simulink model "QPSK_ad9361_radioIO_capture"  (R2017b)
settings: Solver=VariableStepAuto  StartTime=0.0  StopTime=inf  RelTol=1e-3  EnableMultiTasking=on
PreLoadFcn:
  | adi9361_preload(bdroot,'rx');
  | sdrqpsktx = sdrzqpsktxFMC234_init;
  | % sdrqpskrx = sdrzqpskrxFMC234_init;
  | sdrqpskrx = zynqRadioQPSKRxAD9361AD9364SL_init_2MSPS
InitFcn:
  | sdrqpsktx = sdrzqpsktxFMC234_init;
  | % sdrqpskrx = sdrzqpskrxFMC234_init;
  | sdrqpskrx = zynqRadioQPSKRxAD9361AD9364SL_init_2MSPS
undefined symbols (not defined in the file or in its folder): D, dBval, DCLeak_Matrix, designMultirateFIR, dfilt, fuzz_val, GainImb_Matrix, gcbh, IP2_Matrix, IP3_Matrix, magnitude, rcfiltgaincompat
libraries: simrfV2elements x12, simulink x7, dsparch4 x6, simrfV2util1 x4, fl_lib x4, dspmlti4 x3, simrfV2junction1 x3, commdigbbndpm3 x3, dspstat3 x3, dspobslib x3, simulink_extras x2, dspsigattribs x2
(part 2 of 3)

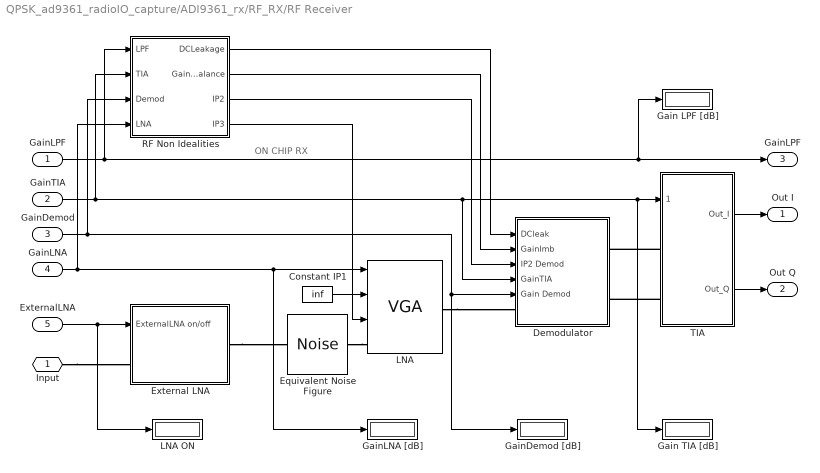
== system QPSK_ad9361_radioIO_capture/ADI9361_rx/RF_RX/RF Receiver ==
  note: ON CHIP RX
  GainLPF : Inport
  GainTIA : Inport  Port=2
  GainDemod : Inport  Port=3
  GainLNA : Inport  Port=4
  ExternalLNA : Inport  Port=5
  Constant IP1 : Constant  Value=inf
  Demodulator : Subsystem
  Equivalent Noise Figure : simrfV2sources1/Noise  SimulinkInputSignalType=Ideal voltage  NoiseType=White  NoisePSD=4*1.381e-23*290*50*10^(NF/10)  CarrierFreq=fc_RF Hz  InternalGrounding=off
      settings: SourceProductName=RF Blockset  SourceProductBaseCode=RB
  External LNA : Subsystem
  Gain LPF [dB] : Display
  Gain TIA [dB] : Display
  GainDemod [dB] : Display
  GainLNA [dB] : Display
  LNA : simrfV2elements/VGA  classname=vga  Zin=Rin  Zout=50  IO=Input  InternalGrounding=on
      settings: SourceProductName=RF Blockset  SourceProductBaseCode=RB
  LNA ON : Display
  RF Non Idealities : Subsystem
  TIA : Subsystem
  Input : PMIOPort  Port=1  Side=Left
  Out I : Outport
  Out Q : Outport  Port=2
  "GainLPF " : Outport  Port=3
  wires:
  GainTIA/1 -> RF Non Idealities/2(TIA), Gain TIA [dB]/1, TIA/1(Gain TIA), Demodulator/4(GainTIA)
  TIA/1(Out_I) -> Out I/1
  TIA/2(Out_Q) -> Out Q/1
  GainDemod/1 -> RF Non Idealities/3(Demod), Demodulator/5(Gain Demod), GainDemod [dB]/1
  GainLNA/1 -> LNA/1, GainLNA [dB]/1, RF Non Idealities/4(LNA)
  GainLPF/1 -> "GainLPF "/1, Gain LPF [dB]/1, RF Non Idealities/1(LPF)
  RF Non Idealities/1(DCLeakage) -> Demodulator/1(DCleak)
  RF Non Idealities/3(IP2) -> Demodulator/3(IP2 Demod)
  RF Non Idealities/4(IP3) -> LNA/3
  Constant IP1/1 -> LNA/2
  ExternalLNA/1 -> LNA ON/1, External LNA/1(ExternalLNA on/off)
  RF Non Idealities/2(GainImbalance) -> Demodulator/2(GainImb)
  connections:
  LNA/RConn1 -- Demodulator/LConn1
  TIA/LConn1 -- Demodulator/RConn1
  TIA/LConn2 -- Demodulator/RConn2
  Equivalent Noise Figure/LConn1 -- LNA/LConn1
  Input/RConn1 -- External LNA/LConn1
  External LNA/RConn1 -- Equivalent Noise Figure/RConn1

== system QPSK_ad9361_radioIO_capture/ADI9361_rx/Subsystem6/Subsystem1 ==
  Data Type Conversion : DataTypeConversion  OutDataTypeStr=boolean
  Pulse Generator2 : DiscretePulseGenerator  SampleTime=Trf
  START : Outport
  wires:
  Pulse Generator2/1 -> Data Type Conversion/1
  Data Type Conversion/1 -> START/1

== system QPSK_ad9361_radioIO_capture/ADI9361_rx/Subsystem6/Subsystem2 ==
  s : Inport
  w : Inport  Port=2
  Data Type Conversion : DataTypeConversion  OutDataTypeStr=boolean
  Subtract1 : Sum  Inputs=-+  OutDataTypeStr=int8
  os : Outport
  ow : Outport  Port=2
  wires:
  s/1 -> Subtract1/2, os/1
  Data Type Conversion/1 -> ow/1
  Subtract1/1 -> Data Type Conversion/1
  w/1 -> Subtract1/1

== system QPSK_ad9361_radioIO_capture/ADI9361_rx/Subsystem6/Subsystem3 ==
  w : Inport
  s : Inport  Port=2
  Data Type Conversion : DataTypeConversion  OutDataTypeStr=boolean
  Subtract1 : Sum  Inputs=-+  OutDataTypeStr=int8
  ow : Outport
  os : Outport  Port=2
  wires:
  w/1 -> Subtract1/1
  Subtract1/1 -> Data Type Conversion/1
  Data Type Conversion/1 -> ow/1
  s/1 -> Subtract1/2, os/1

== system QPSK_ad9361_radioIO_capture/ADI9361_rx/Subsystem6/Wblk4 ==
  Win : Inport
  Sin : Inport  Port=2
  Combinatorial Logic : CombinatorialLogic  TruthTable=[0; 0; 1; 0]
  Mux : Mux  Inputs=2
  Wout : Outport
  wires:
  Mux/1 -> Combinatorial Logic/1
  Combinatorial Logic/1 -> Wout/1  "wout"
  Win/1 -> Mux/1
  Sin/1 -> Mux/2

== system QPSK_ad9361_radioIO_capture/ADI9361_rx/Subsystem6/Wblk4a ==
  Win : Inport
  Sin : Inport  Port=2
  Combinatorial Logic : CombinatorialLogic  TruthTable=[0; 0; 1; 0]
  Mux : Mux  Inputs=2
  Wout : Outport
  wires:
  Mux/1 -> Combinatorial Logic/1
  Combinatorial Logic/1 -> Wout/1  "wout"
  Win/1 -> Mux/1
  Sin/1 -> Mux/2

== system QPSK_ad9361_radioIO_capture/ADI9361_rx/Subsystem6/Wblk5 ==
  Win : Inport
  Sin : Inport  Port=2
  Combinatorial Logic : CombinatorialLogic  TruthTable=[0; 0; 1; 0]
  Mux : Mux  Inputs=2
  Wout : Outport
  wires:
  Mux/1 -> Combinatorial Logic/1
  Combinatorial Logic/1 -> Wout/1  "wout"
  Win/1 -> Mux/1
  Sin/1 -> Mux/2

== system QPSK_ad9361_radioIO_capture/ADI9361_rx/Subsystem6/Wblk6 ==
  Win : Inport
  Sin : Inport  Port=2
  Combinatorial Logic : CombinatorialLogic  TruthTable=[0; 0; 1; 0]
  Mux : Mux  Inputs=2
  Wout : Outport
  wires:
  Mux/1 -> Combinatorial Logic/1
  Combinatorial Logic/1 -> Wout/1  "wout"
  Win/1 -> Mux/1
  Sin/1 -> Mux/2

== system QPSK_ad9361_radioIO_capture/ADI9361_rx/Subsystem6/Wblk7 ==
  Win : Inport
  Sin : Inport  Port=2
  Combinatorial Logic : CombinatorialLogic  TruthTable=[0; 0; 1; 0]
  Mux : Mux  Inputs=2
  Wout : Outport
  wires:
  Mux/1 -> Combinatorial Logic/1
  Combinatorial Logic/1 -> Wout/1  "wout"
  Win/1 -> Mux/1
  Sin/1 -> Mux/2

== system QPSK_ad9361_radioIO_capture/QPSK Receiver1/Coarse Frequency Compensation/Find Frequency Offset ==
  note: Algorithm:
      | 1.  Introduce nonlinearity to create tone at M*Foffset, where M is modulation order
      | 2.  Find index of tone within FFT vector
      | 3.  Compute frequency offset
  In : Inport
  Alphabet size : Constant  Value=M  OutDataTypeStr=Inherit: Inherit via back propagation
  Complex Power : commblksprivate/Complex Power
      settings: SourceProductName=Communications System Toolbox  SourceProductBaseCode=CM
  Find Frequency Offset : MATLAB Function  TreatAsAtomicUnit=on
  Periodogram : dspspect3/Periodogram  measurement=Power spectral density  wintype=Hamming  Rs=50  beta=5  winsamp=Symmetric  FFTImplementation=Auto  inheritFFT=off  fftsize=2048  navg=16  inheritTs=on  Ts=1
      settings: SourceProductName=DSP System Toolbox  SourceProductBaseCode=DS
  Probe : Probe  ProbeComplexSignal=off
  Frq : Outport
  wires:
  Periodogram/1 -> Find Frequency Offset/3(FFTSig)
  Alphabet size/1 -> Complex Power/2
  In/1 -> Complex Power/1
  Probe/1 -> Find Frequency Offset/1(N)
  Probe/2 -> Find Frequency Offset/2(Tf)
  Find Frequency Offset/1(FreqOffset) -> Frq/1
  Complex Power/1 -> Probe/1, Periodogram/1

== system QPSK_ad9361_radioIO_capture/QPSK Receiver1/Data Decoding/Barker Code Symbol Generation  ==
  note: Regenerate a QPSK-modulated unipolar Barker code sequence
      | to be compared with the received data
  Constant Barker Code : Constant  Value=|  VectorParams1D=off
      | [+1 +1 +1 +1 +1 -1 -1 +1 +1 -1 +1 -1 +1
      | ].' > 0
      settings: SamplingMode=Frame based
  Data Type Conversion : DataTypeConversion  OutDataTypeStr=double
  QPSK Modulator Baseband : commdigbbndpm3/QPSK Modulator Baseband  InType=Bit  Enc=Gray  Ph=pi/4  outDtype=double  outWordLen=16  outUDDataType=sfix(16)  outFracLenMode=Best precision  outFracLen=15  outDataTypeStr=double  outLastDataTypeStr=double
  Repeat : dspsigops/Repeat  N=2  InputProcessing=Columns as channels (frame based)  RateOptions=Enforce single-rate processing  ic=0  mode=Unused parameter value
      settings: SourceProductName=DSP System Toolbox
  Out : Outport
  wires:
  Constant Barker Code/1 -> Data Type Conversion/1
  Repeat/1 -> QPSK Modulator Baseband/1
  QPSK Modulator Baseband/1 -> Out/1
  Data Type Conversion/1 -> Repeat/1

== system QPSK_ad9361_radioIO_capture/QPSK Receiver1/Data Decoding/Compute Delay ==
  note: Correlation with the modulated symbols
  Barker Reference : Inport
  Data : Inport  Port=2
  Abs : Abs
  Constant1 : Constant  VectorParams1D=off  OutDataTypeStr=Inherit: Inherit via back propagation  FramePeriod=2
  Correlation : dspstat3/Correlation  domain=Time  roundingMode=Floor  overflowMode=off  accumDataTypeStr=Inherit: Same as product output  accumLastDataTypeStr=Inherit: Same as product output  outputDataTypeStr=Inherit: Same as accumulator  outputMin=[]  outputMax=[]  outputLastDataTypeStr=Inherit: Same as accumulator
      settings: SourceProductName=DSP System Toolbox  SourceProductBaseCode=DS
  Math Function : Math  Operator=mod  SaturateOnIntegerOverflow=on
  Maximum : dspstat3/Maximum  operation=maximum  fcn=Index  indexBase=One  operateOver=Each column  Dimension=1  InputProcessing=Columns as channels (frame based)  reset=None  roiEnable=off  roiType=Rectangles  roiPortion=Entire ROI  roiOutput=Individual statistics for each ROI  roiFlag=off  roundingMode=Floor  overflowMode=off  accumDataTypeStr=Inherit: Same as product output  accumLastDataTypeStr=Inherit: Same as product output
  Probe : Probe  ProbeSampleTime=off  ProbeComplexSignal=off
  Sum : Sum  Inputs=|-+  SaturateOnIntegerOverflow=on  InputSameDT=on  OutDataTypeStr=Inherit: Same as first input
  Sum1 : Sum  Inputs=|+-  SaturateOnIntegerOverflow=on  InputSameDT=on  OutDataTypeStr=Inherit: Same as first input
  Delay : Outport
  wires:
  Abs/1 -> Maximum/1
  Constant1/1 -> Sum1/2
  Sum1/1 -> Math Function/2
  Math Function/1 -> Delay/1
  Sum/1 -> Math Function/1
  Probe/1 -> Sum1/1, Sum/2
  Correlation/1 -> Abs/1
  Maximum/1 -> Sum/1
  Barker Reference/1 -> Correlation/1
  Data/1 -> Correlation/2, Probe/1

== system QPSK_ad9361_radioIO_capture/QPSK Receiver1/Data Decoding/Descrambling ==
  In : Inport
  Descrambler : commsequence2/Descrambler  M=2  poly=[1 1 1 0 1]  iniStaSource=Dialog Parameter  ini_sta=[0 0 0 0]  resetViaPort=off
      settings: SourceProductName=Communications System Toolbox  SourceProductBaseCode=CM
  Selector : Selector  IndexOptions=Index vector (dialog)  Indices=[sdrqpskrx.BarkerLength*log2(sdrqpskrx.M)+1:sdrqpskrx.FrameSize*log2(sdrqpskrx.M)]  OutputSizes=1
  Selector1 : Selector  IndexOptions=Index vector (dialog)  Indices=[1:sdrqpskrx.MsgLength]  OutputSizes=1
  Out : Outport
  wires:
  Descrambler/1 -> Selector1/1
  Selector1/1 -> Out/1
  In/1 -> Selector/1
  Selector/1 -> Descrambler/1

== system QPSK_ad9361_radioIO_capture/QPSK Receiver1/Data Decoding/Phase Ambiguity Correction & Demodulation ==
  note: Phase Ambiguity Resolution
      | and Demodulation
  Phase : Inport
  Data : Inport  Port=2
  Complex Phase Shift : commutil2/Complex Phase Shift
      settings: SourceProductName=Communications System Toolbox  SourceProductBaseCode=CM
  Constellation Diagram RX : ConstellationDiagram
  Gain : Gain  Gain=-1
  QPSK Demodulator Baseband : commdigbbndpm3/QPSK Demodulator Baseband  OutType=Bit  DecType=Hard decision  VarSource=Dialog  Variance=1  Dec=Gray  Ph=pi/4  outDtype1=Inherit via internal rule  outDtype2=Inherit via internal rule  derotateFactorWordLen=16  derotateFactorDataTypeStr=Inherit: Same word length as input  derotateFactorLastDataTypeStr=Inherit: Same word length as input
  Out : Outport
  wires:
  Phase/1 -> Gain/1
  Data/1 -> Complex Phase Shift/1
  Complex Phase Shift/1 -> Constellation Diagram RX/1, QPSK Demodulator Baseband/1
  QPSK Demodulator Baseband/1 -> Out/1
  Gain/1 -> Complex Phase Shift/2

== system QPSK_ad9361_radioIO_capture/QPSK Receiver1/Data Decoding/Phase Offset Estimator ==
  note: 1. The original signal is expressed as y(t) = x(t)e^{j\phi}+n(t), t = 1, 2, ..., N
      | 2. y_1(t) = x{*}(t)y(t) = e^{j\phi} + x{*}(t)n(t)
      | The goal is to estimate the value \phi from the observation y_1(t), t = 1, 2, ...N
      | i.e., estimate the value B = e^{j\phi}, and \phi = angle(B)
      | 3. Suppose n(t) yields to a i.i.d. complex AWGN distribution N(0,\sigma^2).
      | Then a non-biased estimator could be
      | B_{est} = 1/N*sum(y_1(1:N)), and \phi_{est} = angle(B_{est})
      | and the variance of B_{est} is \sigma^2/N
  BarkerRef : Inport
  Data : Inport  Port=2
  Complex to Magnitude-Angle : ComplexToMagnitudeAngle  Output=Angle
  Math Function : Math  Operator=conj  SaturateOnIntegerOverflow=on
  Mean : dspstat3/Mean  run=off  reset_popup=None  InputProcessing=Columns as channels (frame based)  directionMode=Each column  dimension=1  roiEnable=off  roiType=Rectangles  roiPortion=Entire ROI  roiOutput=Individual statistics for each ROI  roiFlag=off  outputDataTypeStr=Inherit: Same as accumulator  outputLastDataTypeStr=Inherit: Same as accumulator  outputMin=[]  outputMax=[]  roundingMode=Floor  overflowMode=off
  Phase Offset Detection : MATLAB Function  TreatAsAtomicUnit=on
  Product : Product  RndMeth=Zero
  Selector : Selector  IndexOptions=Index vector (dialog)  Indices=[1:sdrqpskrx.BarkerLength]  OutputSizes=1
  Phase : Outport
  wires:
  Data/1 -> Selector/1
  BarkerRef/1 -> Math Function/1  "x(t)"
  Selector/1 -> Product/2  "y(t)"
  Math Function/1 -> Product/1  "x*(t)"
  Product/1 -> Mean/1  "y_1(t)"
  Mean/1 -> Complex to Magnitude-Angle/1
  Complex to Magnitude-Angle/1 -> Phase Offset Detection/1(In)
  Phase Offset Detection/1(Out) -> Phase/1

== system QPSK_ad9361_radioIO_capture/QPSK Receiver1/Fine Frequency Compensation/DDS ==
  note: The digital filter acts as a pure integrator
  In : Inport
  Digital Filter : dspobslib/Digital Filter  TypePopup=IIR (poles & zeros)  IIRFiltStruct=Direct form II transposed  AllPoleFiltStruct=Direct form  FIRFiltStruct=Direct form  CoeffSource=Specify via dialog  NumCoeffs=[0 1]  DenCoeffs=[1 -1]  BiQuadCoeffs=[1 0.3 0.4 1 0.1 0.2]  LatticeCoeffs=[0.2 0.4]  denIgnore=on  FiltPerSampPopup=One filter per frame  IC=0  ICnum=0  ICden=0  roundingMode=Floor  overflowMode=off  ScaleValues=1  scaleValueFracLength=14  stageInFracLength=15  stageOutFracLength=15  FilterSource=Specify via dialog  dfiltObjectName=dfilt.dffir([1 2 1])  InputProcessing=Columns as channels (frame based)
      settings: SourceProductName=DSP System Toolbox  SourceProductBaseCode=DS
  Gain : Gain  Gain=-1*sdrqpskrx.FineFreqCompensateGain
  Phase : Outport
  wires:
  Digital Filter/1 -> Gain/1
  In/1 -> Digital Filter/1
  Gain/1 -> Phase/1

== system QPSK_ad9361_radioIO_capture/QPSK Receiver1/Fine Frequency Compensation/Loop Filter ==
  note: Proportional-plus-Integrator Loop Filter,
      | Infinite DC Response to guarantee convergence
  e : Inport
  Digital Filter : dspobslib/Digital Filter  TypePopup=IIR (poles & zeros)  IIRFiltStruct=Direct form II transposed  AllPoleFiltStruct=Direct form  FIRFiltStruct=Direct form  CoeffSource=Specify via dialog  NumCoeffs=[1 0]  DenCoeffs=[1 -1]  BiQuadCoeffs=[1 0.3 0.4 1 0.1 0.2]  LatticeCoeffs=[0.2 0.4]  denIgnore=on  FiltPerSampPopup=One filter per frame  IC=0  ICnum=0  ICden=0  roundingMode=Floor  overflowMode=off  ScaleValues=1  scaleValueFracLength=14  stageInFracLength=15  stageOutFracLength=15  FilterSource=Specify via dialog  dfiltObjectName=dfilt.dffir([1 2 1])  InputProcessing=Columns as channels (frame based)
      settings: SourceProductName=DSP System Toolbox  SourceProductBaseCode=DS
  K1 : Gain  Gain=K1
  K2 : Gain  Gain=K2
  Sum2 : Sum  SaturateOnIntegerOverflow=on  InputSameDT=on  OutDataTypeStr=Inherit: Same as first input
  v : Outport
  wires:
  K2/1 -> Digital Filter/1
  Digital Filter/1 -> Sum2/2
  Sum2/1 -> v/1
  e/1 -> K2/1, K1/1
  K1/1 -> Sum2/1

== system QPSK_ad9361_radioIO_capture/QPSK Receiver1/Timing Recovery/Modified Buffer ==
  Data : Inport
  Clk : Inport  Port=2
  Logical Operator : Logic  AllPortsSameDT=off  OutDataTypeStr=boolean
  Modified Buffer : Subsystem
  DataOut : Outport
  DataValid : Outport  Port=2
  wires:
  Data/1 -> Modified Buffer/1(In1)
  Clk/1 -> Modified Buffer/Enable, Logical Operator/2
  Modified Buffer/1(DataOut) -> DataOut/1
  Modified Buffer/2(DataValid) -> Logical Operator/1
  Logical Operator/1 -> DataValid/1

== system QPSK_ad9361_radioIO_capture/QPSK Receiver1/Timing Recovery/Timing Recovery PLL ==
  note: Sample-based processing is adopted because
      | 1. Strobe signal is required to generate for EVERY sample for processing and output
      | sampling, delayed strobe signal would affect the accuracy of bit stripping/stuffing
      | 2. The BER performance degrades significantly even with frame size 2 and 4
  note: Baseband implementation of the Symbol Timing Synchronization listed in Chapter 8.4
      | of "Digital Communications- A Discrete-Time Approach" by Michael Rice. See Appendix
      | C.2 of the same book for the details of PLL design.
  note: To determine phase error detector gain K_p, See Equation 8.42 &
      | Figure 8.4.7 of "Digital Communications - A Discrete-Time Approach"
      | by Michael Rice.
  DataIn : Inport
  Integer Delay1 : Delay  DelayLength=1  InputProcessing=Inherited
  Integer Delay2 : Delay  DelayLength=1  InputProcessing=Inherited
  Interpolation Filter : MATLAB Function  TreatAsAtomicUnit=on
  Loop Filter : Subsystem  mask{BnTs=0.01, zeta=1, Kp=sdrqpskrx.TimingRecTEDGain, K0=sdrqpskrx.TimingRecCompensateGain, N=sdrqpskrx.Upsampling/sdrqpskrx.Downsampling}
      mask prompts: BnTs "Loop Bandwidth"; zeta "Loop Damping Factor"; Kp "Phase Detector Gain (Kp)"; K0 "DDS gain (K0)"; N "Number of Samples/symbol (N)"
      mask init:
      | % See C.57 to C.61 in Michael Rice's "Digital Communications 
      | % - A Discrete-Time Approach" for details
      | theta = BnTs/(zeta+0.25/zeta)/N;
      | d = 1 + 2*zeta*theta + theta*theta;
      | K1 = 4*zeta*theta/d;
      | K2 = 4*theta*theta/d;
      | K1 = K1/(Kp*K0);
      | K2 = K2/(Kp*K0);
      mask Display: disp('Loop Filter');
  NCO Control : MATLAB Function
  Timing Error Detector : MATLAB Function  TreatAsAtomicUnit=on
  DataOut : Outport
  ClkOut : Outport  Port=2
  wires:
  DataIn/1 -> Interpolation Filter/1(In)
  NCO Control/2(mu) -> Integer Delay2/1
  Integer Delay1/1 -> ClkOut/1, Timing Error Detector/2(strobe)
  NCO Control/1(Underflow) -> Integer Delay1/1
  Interpolation Filter/1(Out) -> DataOut/1, Timing Error Detector/1(In)
  Loop Filter/1(v) -> NCO Control/1(Delta)
  Timing Error Detector/1(e) -> Loop Filter/1(e)
  Integer Delay2/1 -> Interpolation Filter/2(mu)

== system QPSK_ad9361_radioIO_capture/QPSK TX/Bit Generation/Barker Code SS ==
  Constant Barker Code : Constant  Value=|  VectorParams1D=off
      | [+1 +1 +1 +1 +1 -1 -1 +1 +1 -1 +1 -1 +1
      | ].' > 0  % Bipolar to Unipolar Conversion
      settings: SamplingMode=Frame based
  Data Type Conversion : DataTypeConversion  OutDataTypeStr=double
  Out : Outport
  wires:
  Data Type Conversion/1 -> Out/1
  Constant Barker Code/1 -> Data Type Conversion/1

== system QPSK_ad9361_radioIO_capture/QPSK TX/Bit Generation/Message Source ==
  Bernoulli Binary Generator : commrandsrc2/Bernoulli Binary Generator  P=0.5  seed=61  Ts=sdrqpsktx.FrameTime/(sdrqpsktx.DataLength-sdrqpsktx.MsgLength)  frameBased=on  sampPerFrame=sdrqpsktx.DataLength-sdrqpsktx.MsgLength  orient=off  outDataType=double
  Matrix Concatenate : Concatenate  Mode=Multidimensional array
  Message Generator : MATLAB Function  TreatAsAtomicUnit=on
  Out : Outport
  wires:
  Matrix Concatenate/1 -> Out/1
  Bernoulli Binary Generator/1 -> Matrix Concatenate/2
  Message Generator/1(msg) -> Matrix Concatenate/1

== system QPSK_ad9361_radioIO_capture/ADI9361_rx/ADC_RX/ADC_I/Quantizer1 ==
  u : Inport
  Abs : Abs
  Idealized ADC quantizer : simulink_extras/Additional Discrete/Idealized ADC quantizer  NumberOfConverterBits=3  Vmin=0  Vmax=.8  OutputDataType=double  OutputNegativeValues=off
      settings: SourceProductName=Simulink
  Product : Product
  Saturation : Saturate  UpperLimit=0.41
  Sign : Signum
  y : Outport
  wires:
  u/1 -> Sign/1, Abs/1
  Saturation/1 -> Idealized ADC quantizer/1
  Idealized ADC quantizer/1 -> Product/1
  Sign/1 -> Product/2
  Abs/1 -> Saturation/1
  Product/1 -> y/1

== system QPSK_ad9361_radioIO_capture/ADI9361_rx/ADC_RX/ADC_Q/Quantizer1 ==
  u : Inport
  Abs : Abs
  Idealized ADC quantizer : simulink_extras/Additional Discrete/Idealized ADC quantizer  NumberOfConverterBits=3  Vmin=0  Vmax=.8  OutputDataType=double  OutputNegativeValues=off
      settings: SourceProductName=Simulink
  Product : Product
  Saturation : Saturate  UpperLimit=0.41
  Sign : Signum
  y : Outport
  wires:
  u/1 -> Sign/1, Abs/1
  Saturation/1 -> Idealized ADC quantizer/1
  Idealized ADC quantizer/1 -> Product/1
  Sign/1 -> Product/2
  Abs/1 -> Saturation/1
  Product/1 -> y/1

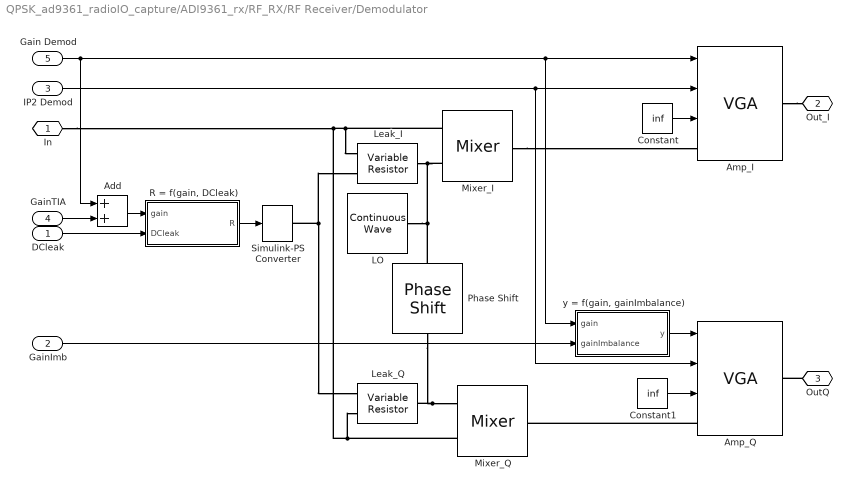
== system QPSK_ad9361_radioIO_capture/ADI9361_rx/RF_RX/RF Receiver/Demodulator ==
  DCleak : Inport
  GainImb : Inport  Port=2
  IP2 Demod : Inport  Port=3
  GainTIA : Inport  Port=4
  Gain Demod : Inport  Port=5
  Add : Sum
  Amp_I : simrfV2elements/VGA  classname=vga  Zin=100  Zout=100  IO=Input  InternalGrounding=on
      settings: SourceProductName=RF Blockset  SourceProductBaseCode=RB
  Amp_Q : simrfV2elements/VGA  classname=vga  Zin=100  Zout=100  IO=Input  InternalGrounding=on
      settings: SourceProductName=RF Blockset  SourceProductBaseCode=RB
  Constant : Constant  Value=inf
  Constant1 : Constant  Value=inf
  LO : simrfV2sources1/Continuous Wave  CWSourceType=Ideal voltage  Z0=0  IVoltage=1/sqrt(2) V  ICurrent=0 A  MagPower=1 W  QVoltage=0 V  QCurrent=0 A  AnglePower=0  CarrierFreq=RF Hz  InternalGrounding=on
      settings: SourceProductName=RF Blockset  SourceProductBaseCode=RB
  Leak_I : fl_lib/Electrical/Electrical Elements/Variable Resistor  Rmin=0 Ohm  i_specify=off  i_priority=High  i=0 A  v_specify=off  v_priority=High  v=0 V
  Leak_Q : fl_lib/Electrical/Electrical Elements/Variable Resistor  Rmin=0 Ohm  i_specify=off  i_priority=High  i=0 A  v_specify=off  v_priority=High  v=0 V
  Mixer_I : simrfV2elements/Mixer  classname=mixer  Source_linear_gain=Available power gain  linear_gain=0 dB  Zin=100  Zout=100  ZLO=inf  Source_Poly=Even and odd order  Poly_Coeffs=[0 1]  IPType=Output  IP2=Inf dBm  IP3=Inf dBm  P1dB=Inf dBm  Psat=Inf dBm  Gcomp=Inf dBm  NF=0  InternalGrounding=on
      settings: SourceProductName=RF Blockset  SourceProductBaseCode=RB
  Mixer_Q : simrfV2elements/Mixer  classname=mixer  Source_linear_gain=Available power gain  linear_gain=0 dB  Zin=100  Zout=100  ZLO=inf  Source_Poly=Even and odd order  Poly_Coeffs=[0 1]  IPType=Output  IP2=Inf dBm  IP3=Inf dBm  P1dB=Inf dBm  Psat=Inf dBm  Gcomp=Inf dBm  NF=0  InternalGrounding=on
      settings: SourceProductName=RF Blockset  SourceProductBaseCode=RB
  Phase Shift : simrfV2elements/Phase Shift  PhaseShift=90 deg  InternalGrounding=on
      settings: SourceProductName=RF Blockset  SourceProductBaseCode=RB
  "R = f(gain, DCleak)" : Subsystem
  Simulink-PS Converter : nesl_utility/Simulink-PS Converter  PhysicalDomain=network_engine_domain  SubClassName=ps_input  LeftPortType=input  RightPortType=output  PseudoPeriodic=off  Frequencies=[]  NoiseDistribution=none  NoiseParameters=[]  Unit=1  AffineConversion=off  InputFiltering=off  SimscapeFilterOrder=1  InputFilterTimeConstant=0.001  UdotUserProvided=1
  "y = f(gain, gainImbalance)" : Subsystem
  In : PMIOPort  Port=1  Side=Left
  Out_I : PMIOPort  Port=2  Side=Right
  OutQ : PMIOPort  Port=3  Side=Right
  wires:
  Gain Demod/1 -> "y = f(gain, gainImbalance)"/1(gain), Amp_I/1, Add/1
  IP2 Demod/1 -> Amp_Q/2, Amp_I/2
  "R = f(gain, DCleak)"/1(R) -> Simulink-PS Converter/1
  GainTIA/1 -> Add/2
  Add/1 -> "R = f(gain, DCleak)"/1(gain)
  GainImb/1 -> "y = f(gain, gainImbalance)"/2(gainImbalance)
  DCleak/1 -> "R = f(gain, DCleak)"/2(DCleak)
  "y = f(gain, gainImbalance)"/1(y) -> Amp_Q/1
  Constant/1 -> Amp_I/3
  Constant1/1 -> Amp_Q/3
  connections:
  Phase Shift/RConn1 -- Mixer_Q/LConn2 -- Leak_Q/RConn1
  Mixer_I/LConn2 -- Leak_I/RConn1 -- LO/LConn1 -- Phase Shift/LConn1
  Mixer_Q/LConn1 -- Leak_Q/LConn2 -- In/RConn1 -- Leak_I/LConn2 -- Mixer_I/LConn1
  Amp_I/RConn1 -- Out_I/RConn1
  OutQ/RConn1 -- Amp_Q/RConn1
  Mixer_I/RConn1 -- Amp_I/LConn1
  Amp_Q/LConn1 -- Mixer_Q/RConn1
  Simulink-PS Converter/RConn1 -- Leak_Q/LConn1 -- Leak_I/LConn1

== system QPSK_ad9361_radioIO_capture/ADI9361_rx/RF_RX/RF Receiver/External LNA ==
  ExternalLNA on/off : Inport
  Bypass : simrfV2junction1/Switch  classname=switch  Ron=0 Ohm  Roff=inf Ohm  Vthres=0.5 V
      settings: SourceProductName=RF Blockset  SourceProductBaseCode=RB
  Invert Control : Subsystem
  LNA : simrfV2elements/Amplifier  classname=amplifier  DataSource=Data file  File=simrfV2_unitygain.s2p  Paramtype=S-parameters  Sparam=[0 0;1 0]  SparamFreq=1e9 Hz  SparamZ0=50  Residues=0  Poles=0  DF={0 0; 1 0}  Source_linear_gain=Available power gain  linear_gain=10 dB  Zin=50  Zout=50  Source_Poly=Even and odd order  Poly_Coeffs=[0 1]  IPType=Output  IP2=inf dBm  IP3=inf dBm  P1dB=inf dBm  Psat=inf dBm  Gcomp=inf dBm  NF=0  InternalGrounding=on  SourceFreq=Extracted from data source  PlotFreq=[1e9:1e6:3e9] Hz  PlotType=X-Y plane  YParam1=S11  YFormat1=Magnitude (decibels)  YParam2=None  YFormat2=Magnitude (decibels)  YOption=Linear  XOption=Linear  SparamRepresentation=Time domain (rationalfit)  FitTol=-40  FitOpt=Fit individually  AutoImpulseLength=on  ImpulseLength=1e-10 s
      settings: SourceProductName=RF Blockset  SourceProductBaseCode=RB
  LNA on input : simrfV2junction1/Switch  classname=switch  Ron=0 Ohm  Roff=inf Ohm  Vthres=0.5 V
      settings: SourceProductName=RF Blockset  SourceProductBaseCode=RB
  LNA on ouput : simrfV2junction1/Switch  classname=switch  Ron=0 Ohm  Roff=inf Ohm  Vthres=0.5 V
      settings: SourceProductName=RF Blockset  SourceProductBaseCode=RB
  in : PMIOPort  Port=1  Side=Left
  out : PMIOPort  Port=2  Side=Right
  wires:
  ExternalLNA on/off/1 -> LNA on ouput/1, LNA on input/1, Invert Control/1(In)
  Invert Control/1(Out) -> Bypass/1
  connections:
  Bypass/RConn1 -- out/RConn1 -- LNA on ouput/RConn1
  LNA on input/LConn1 -- Bypass/LConn1 -- in/RConn1
  LNA on input/RConn1 -- LNA/LConn1
  LNA/RConn1 -- LNA on ouput/LConn1

== system QPSK_ad9361_radioIO_capture/ADI9361_rx/RF_RX/RF Receiver/RF Non Idealities ==
  LPF : Inport
  TIA : Inport  Port=2
  Demod : Inport  Port=3
  LNA : Inport  Port=4
  DetectChange : Subsystem
  RF Non Idealities : Subsystem
  DCLeakage : Outport
  GainImbalance : Outport  Port=2
  IP2 : Outport  Port=3
  IP3 : Outport  Port=4
  wires:
  TIA/1 -> RF Non Idealities/3(TIA), DetectChange/3(In3)
  LPF/1 -> RF Non Idealities/4(LPF), DetectChange/4(In4)
  Demod/1 -> RF Non Idealities/2(Demod), DetectChange/2(In2)
  LNA/1 -> RF Non Idealities/1(LNA), DetectChange/1(In1)
  RF Non Idealities/1(DCLeakage) -> DCLeakage/1
  RF Non Idealities/2(GainImbalance) -> GainImbalance/1
  RF Non Idealities/3(IP2) -> IP2/1
  RF Non Idealities/4(IP3) -> IP3/1
  DetectChange/1(Trigger) -> RF Non Idealities/Trigger

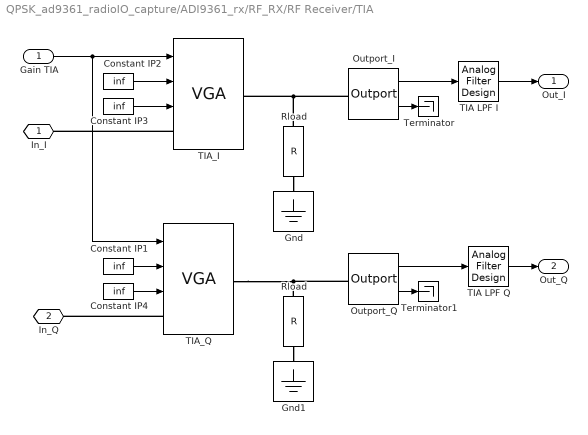
== system QPSK_ad9361_radioIO_capture/ADI9361_rx/RF_RX/RF Receiver/TIA ==
  Gain TIA : Inport
  " Rload" : simrfV2elements/R  classname=resistor  Resistance=100 Ohm  AddNoise=on
      settings: SourceProductName=RF Blockset  SourceProductBaseCode=RB
  Constant IP{1..4} (4 alike) : Constant  Value=inf
  Gnd : fl_lib/Electrical/Electrical Elements/Electrical Reference
  Gnd1 : fl_lib/Electrical/Electrical Elements/Electrical Reference
  Outport_I : simrfV2util1/Outport  SensorType=Ideal voltage  OutputFormat=In-phase and Quadrature Baseband  CarrierFreq=0 Hz  ZL=Inf  InternalGrounding=on  StepSize=-1 s  AutoStep=off
      settings: SourceProductName=RF Blockset  SourceProductBaseCode=RB
  Outport_Q : simrfV2util1/Outport  SensorType=Ideal voltage  OutputFormat=In-phase and Quadrature Baseband  CarrierFreq=0 Hz  ZL=Inf  InternalGrounding=on  StepSize=-1 s  AutoStep=off
      settings: SourceProductName=RF Blockset  SourceProductBaseCode=RB
  Rload : simrfV2elements/R  classname=resistor  Resistance=100 Ohm  AddNoise=on
      settings: SourceProductName=RF Blockset  SourceProductBaseCode=RB
  TIA LPF I : dsparch4/Analog Filter Design  method=Butterworth  filttype=Lowpass  N=1  Wlo=2.5*ad9361_rx_pars.Fpass*2*pi  Whi=80  Rp=2  Rs=40
  TIA LPF Q : dsparch4/Analog Filter Design  method=Butterworth  filttype=Lowpass  N=1  Wlo=2.5*ad9361_rx_pars.Fpass*2*pi  Whi=80  Rp=2  Rs=40
  TIA_I : simrfV2elements/VGA  classname=vga  Zin=100  Zout=100  IO=Input  InternalGrounding=on
      settings: SourceProductName=RF Blockset  SourceProductBaseCode=RB
  TIA_Q : simrfV2elements/VGA  classname=vga  Zin=100  Zout=100  IO=Input  InternalGrounding=on
      settings: SourceProductName=RF Blockset  SourceProductBaseCode=RB
  Terminator : Terminator
  Terminator1 : Terminator
  In_I : PMIOPort  Port=1  Side=Left
  In_Q : PMIOPort  Port=2  Side=Left
  Out_I : Outport
  Out_Q : Outport  Port=2
  wires:
  Outport_Q/1 -> TIA LPF Q/1
  Outport_I/1 -> TIA LPF I/1
  Outport_I/2 -> Terminator/1
  Outport_Q/2 -> Terminator1/1
  Gain TIA/1 -> TIA_Q/1, TIA_I/1
  TIA LPF I/1 -> Out_I/1
  TIA LPF Q/1 -> Out_Q/1
  Constant IP2/1 -> TIA_I/2
  Constant IP3/1 -> TIA_I/3
  Constant IP1/1 -> TIA_Q/2
  Constant IP4/1 -> TIA_Q/3
  connections:
  TIA_I/LConn1 -- In_I/RConn1
  TIA_Q/LConn1 -- In_Q/RConn1
  Outport_I/LConn1 -- Rload/LConn1 -- TIA_I/RConn1
  Outport_Q/LConn1 -- TIA_Q/RConn1 -- " Rload"/LConn1
  Rload/RConn1 -- Gnd/LConn1
  " Rload"/RConn1 -- Gnd1/LConn1

== system QPSK_ad9361_radioIO_capture/QPSK Receiver1/Timing Recovery/Modified Buffer/Modified Buffer ==
  In1 : Inport
  Enable : EnablePort
  Compare To Constant : simulink/Logic and Bit Operations/Compare To Constant  relop===  const=(bufSize-1)  OutDataTypeStr=boolean  ZeroCross=off
  Counter Limited : simulink/Sources/Counter Limited  uplimit=(bufSize-1)  tsamp=-1
  Delay Line : dspbuff3/Delay Line  siz=bufSize  ic=0  directfeed=on  enable_output=on  hold_output=off  OutputFrames=on
      settings: SourceProductName=DSP System Toolbox  SourceProductBaseCode=DS
  DataOut : Outport
  DataValid : Outport  Port=2
  wires:
  Compare To Constant/1 -> Delay Line/2, DataValid/1
  Delay Line/1 -> DataOut/1
  In1/1 -> Delay Line/1
  Counter Limited/1 -> Compare To Constant/1

== system QPSK_ad9361_radioIO_capture/QPSK Receiver1/Timing Recovery/Timing Recovery PLL/Loop Filter ==
  note: Proportional-Plus-Integrator Loop Filter,
      | Infinite DC Response to guarantee convergence
  e : Inport
  Digital Filter : dspobslib/Digital Filter  TypePopup=IIR (poles & zeros)  IIRFiltStruct=Direct form II transposed  AllPoleFiltStruct=Direct form  FIRFiltStruct=Direct form  CoeffSource=Specify via dialog  NumCoeffs=[1 0]  DenCoeffs=[1 -1]  BiQuadCoeffs=[1 0.3 0.4 1 0.1 0.2]  LatticeCoeffs=[0.2 0.4]  denIgnore=on  FiltPerSampPopup=One filter per frame  IC=0  ICnum=0  ICden=0  roundingMode=Floor  overflowMode=off  ScaleValues=1  scaleValueFracLength=14  stageInFracLength=15  stageOutFracLength=15  FilterSource=Specify via dialog  dfiltObjectName=dfilt.dffir([1 2 1])  InputProcessing=Columns as channels (frame based)
      settings: SourceProductName=DSP System Toolbox  SourceProductBaseCode=DS
  K1 : Gain  Gain=K1
  K2 : Gain  Gain=K2
  Sum2 : Sum  SaturateOnIntegerOverflow=on  InputSameDT=on  OutDataTypeStr=Inherit: Same as first input
  v : Outport
  wires:
  K2/1 -> Digital Filter/1
  Digital Filter/1 -> Sum2/2
  Sum2/1 -> v/1
  e/1 -> K2/1, K1/1
  K1/1 -> Sum2/1

== system QPSK_ad9361_radioIO_capture/ADI9361_rx/RF_RX/RF Receiver/Demodulator/R = f(gain, DCleak) ==
  gain : Inport
  DCleak : Inport  Port=2
  Add : Sum  Inputs=--+-+
  Add1 : Sum  Inputs=+-
  Constant1 : Constant  Value=20
  Constant2 : Constant  Value=27
  Constant3 : Constant  Value=3
  Constant4 : Constant  Value=25
  Gain1 : Gain  Gain=(-1)/20
  Gain2 : Gain  Gain=25
  expon3 : Math  Operator=10^u  SaturateOnIntegerOverflow=on
  R : Outport
  wires:
  Add1/1 -> R/1
  Constant4/1 -> Add1/2
  Gain2/1 -> Add1/1
  Gain1/1 -> expon3/1
  Constant2/1 -> Add/4
  Constant1/1 -> Add/3
  Constant3/1 -> Add/2
  DCleak/1 -> Add/5
  Add/1 -> Gain1/1
  gain/1 -> Add/1
  expon3/1 -> Gain2/1

== system QPSK_ad9361_radioIO_capture/ADI9361_rx/RF_RX/RF Receiver/Demodulator/y = f(gain, gainImbalance) ==
  gain : Inport
  gainImbalance : Inport  Port=2
  Add2 : Sum
  Constant2 : Constant  Value=2
  Gain4 : Gain  Gain=1/20
  Gain5 : Gain  Gain=1/20
  Gain6 : Gain  Gain=20
  Times1 : Product  Inputs=***
  expon2 : Math  Operator=10^u  SaturateOnIntegerOverflow=on
  expon3 : Math  Operator=10^u  SaturateOnIntegerOverflow=on
  log1 : Math  Operator=log10  SaturateOnIntegerOverflow=on
  y : Outport
  wires:
  expon2/1 -> Times1/2
  Gain5/1 -> expon3/1
  Times1/1 -> Add2/2
  Gain4/1 -> expon2/1
  Add2/1 -> log1/1
  log1/1 -> Gain6/1
  gain/1 -> Gain5/1
  expon3/1 -> Times1/1, Add2/1
  gainImbalance/1 -> Gain4/1
  Constant2/1 -> Times1/3
  Gain6/1 -> y/1

== system QPSK_ad9361_radioIO_capture/ADI9361_rx/RF_RX/RF Receiver/External LNA/Invert Control ==
  In : Inport
  Data Type Conversion : DataTypeConversion  OutDataTypeStr=boolean
  Data Type Conversion1 : DataTypeConversion  OutDataTypeStr=double
  Logical Operator : Logic  Operator=NOT  AllPortsSameDT=off  OutDataTypeStr=boolean
  Out : Outport
  wires:
  In/1 -> Data Type Conversion/1
  Logical Operator/1 -> Data Type Conversion1/1
  Data Type Conversion/1 -> Logical Operator/1
  Data Type Conversion1/1 -> Out/1

== system QPSK_ad9361_radioIO_capture/ADI9361_rx/RF_RX/RF Receiver/RF Non Idealities/DetectChange ==
  In1 : Inport
  In2 : Inport  Port=2
  In3 : Inport  Port=3
  In4 : Inport  Port=4
  Detect Change{,1..4} (5 alike) : simulink/Logic and Bit Operations/Detect Change  vinit=0  InputProcessing=Inherited  OutDataTypeStr=boolean
  Logical Operator : Logic  Operator=OR  Inputs=5  AllPortsSameDT=off  OutDataTypeStr=boolean
  Step : Step  Time=2*Tstep  SampleTime=Tstep  VectorParams1D=off  ZeroCross=off
  Trigger : Outport
  wires:
  Detect Change/1 -> Logical Operator/4
  Detect Change1/1 -> Logical Operator/3
  Detect Change2/1 -> Logical Operator/2
  In4/1 -> Detect Change3/1
  In2/1 -> Detect Change1/1
  In3/1 -> Detect Change2/1
  Detect Change3/1 -> Logical Operator/1
  In1/1 -> Detect Change/1
  Logical Operator/1 -> Trigger/1
  Detect Change4/1 -> Logical Operator/5
  Step/1 -> Detect Change4/1

== system QPSK_ad9361_radioIO_capture/ADI9361_rx/RF_RX/RF Receiver/RF Non Idealities/RF Non Idealities ==
  LNA : Inport
  Demod : Inport  Port=2
  TIA : Inport  Port=3
  LPF : Inport  Port=4
  Trigger : TriggerPort  VariantControl=Variant  PortDimensions=1
  RF NonIdealities : MATLAB Function  TreatAsAtomicUnit=on
      mask init:
      | load ADI9361Tables;
  DCLeakage : Outport
  GainImbalance : Outport  Port=2
  IP2 : Outport  Port=3
  IP3 : Outport  Port=4
  wires:
  RF NonIdealities/1(Leak) -> DCLeakage/1
  RF NonIdealities/2(GainImb) -> GainImbalance/1
  RF NonIdealities/3(IP2) -> IP2/1
  RF NonIdealities/4(IP3) -> IP3/1
  LNA/1 -> RF NonIdealities/1(LNA)
  LPF/1 -> RF NonIdealities/4(LPF)
  Demod/1 -> RF NonIdealities/2(Demod)
  TIA/1 -> RF NonIdealities/3(TIA)

== matlab function QPSK_ad9361_radioIO_capture/QPSK TX/Bit Generation/Message Source/Message Generator ==
  data: msg output
function msg = genMsg
%#codegen
persistent msgStrSet count;
if isempty(msgStrSet)
    count = 0;
    msgStrSet = ['Hello world 000';...
              'Hello world 001';...
              'Hello world 002';...
              'Hello world 003';...
              'Hello world 004';...
              'Hello world 005';...
              'Hello world 006';...
              'Hello world 007';...
              'Hello world 008';...
              'Hello world 009';...
              'Hello world 010';...
              'Hello world 011';...
              'Hello world 012';...
              'Hello world 013';...
              'Hello world 014';...
              'Hello world 015';...
              'Hello world 016';...
              'Hello world 017';...
              'Hello world 018';...
              'Hello world 019';...
              'Hello world 020';...
              'Hello world 021';...
              'Hello world 022';...
              'Hello world 023';...
              'Hello world 024';...
              'Hello world 025';...
              'Hello world 026';...
              'Hello world 027';...
              'Hello world 028';...
              'Hello world 029';...
              'Hello world 030';...
              'Hello world 031';...
              'Hello world 032';...
              'Hello world 033';...
              'Hello world 034';...
              'Hello world 035';...
              'Hello world 036';...
              'Hello world 037';...
              'Hello world 038';...
              'Hello world 039';...
              'Hello world 040';...
              'Hello world 041';...
              'Hello world 042';...
              'Hello world 043';...
              'Hello world 044';...
              'Hello world 045';...
              'Hello world 046';...
              'Hello world 047';...
              'Hello world 048';...
              'Hello world 049';...
              'Hello world 050';...
              'Hello world 051';...
              'Hello world 052';...
              'Hello world 053';...
              'Hello world 054';...
              'Hello world 055';...
              'Hello world 056';...
              'Hello world 057';...
              'Hello world 058';...
              'Hello world 059';...
              'Hello world 060';...
              'Hello world 061';...
              'Hello world 062';...
              'Hello world 063';...
              'Hello world 064';...
              'Hello world 065';...
              'Hello world 066';...
              'Hello world 067';...
              'Hello world 068';...
              'Hello world 069';...
              'Hello world 070';...
              'Hello world 071';...
              'Hello world 072';...
              'Hello world 073';...
              'Hello world 074';...
              'Hello world 075';...
              'Hello world 076';...
              'Hello world 077';...
              'Hello world 078';...
              'Hello world 079';...
              'Hello world 080';...
              'Hello world 081';...
              'Hello world 082';...
              'Hello world 083';...
              'Hello world 084';...
              'Hello world 085';...
              'Hello world 086';...
              'Hello world 087';...
              'Hello world 088';...
              'Hello world 089';...
              'Hello world 090';...
              'Hello world 091';...
              'Hello world 092';...
              'Hello world 093';...
              'Hello world 094';...
              'Hello world 095';...
              'Hello world 096';...
              'Hello world 097';...
              'Hello world 098';...
              'Hello world 099'];              
end
msgStr = msgStrSet(count+1,:);
msgBin = de2bi(int8(msgStr),7,'left-msb');
msg = reshape(double(msgBin).',105,1);
count = mod(count+1,100);

== matlab function QPSK_ad9361_radioIO_capture/ADI9361_rx/RF_RX/RF Receiver/RF Non Idealities/RF Non Idealities/RF NonIdealities ==
  data: LNA input; Leak output; Demod input; TIA input; LPF input; GainImb output; IP2 output; IP3 output; DCLeak_Matrix parameter; GainImb_Matrix parameter; IP3_Matrix parameter; IP2_Matrix parameter
function [Leak, GainImb, IP2, IP3] =                                    ...
    nonIdealsRF(LNA, Demod, TIA, LPF, DCLeak_Matrix, GainImb_Matrix,    ...
    IP3_Matrix, IP2_Matrix)
%#codegen
coder.extrinsic('griddatan','warning');
IP2 = 200;
IP3 = 200;
Leak = -200;
GainImb = -200;
Leak(:) = griddatan(DCLeak_Matrix(:,1:4), DCLeak_Matrix(:,5),           ...
    [LNA, Demod, TIA, LPF]);
GainImb(:) = griddatan(GainImb_Matrix(:,1:4), GainImb_Matrix(:,5),      ...
    [LNA, Demod, TIA, LPF]);
IP2(:) = griddatan(IP2_Matrix(:,1:4), IP2_Matrix(:,5),[LNA,Demod,TIA,LPF]);
IP3(:) = griddatan(IP3_Matrix(:,1:4), IP3_Matrix(:,5),[LNA,Demod,TIA,LPF]);

if isnan(IP2)
    IP2(:) = griddatan(IP2_Matrix(:,1:4), IP2_Matrix(:,5),              ...
        [LNA, Demod, TIA, LPF],'nearest');
    % Warning('Failed interpolation on IP2');
end
if isnan(IP3)
    IP3(:) = griddatan(IP3_Matrix(:,1:4), IP3_Matrix(:,5),              ...
        [LNA, Demod, TIA, LPF],'nearest');
    % Warning('Failed interpolation on IP3');
end
if isnan(Leak)
    Leak(:) = griddatan(DCLeak_Matrix(:,1:4), DCLeak_Matrix(:,5),       ...
        [LNA, Demod, TIA, LPF],'nearest');
    % Warning('Failed interpolation on DC leakage');
end
if isnan(GainImb)
    GainImb(:) = griddatan(GainImb_Matrix(:,1:4), GainImb_Matrix(:,5),  ...
        [LNA, Demod, TIA, LPF],'nearest');
    % Warning('Failed interpolation on Gain Imbalance');
end

IP2 = 2*(IP2+LNA);

== stateflow chart QPSK_ad9361_radioIO_capture/ADI9361_rx/AGC ==
  settings: executeAtInitialization=1
  state InitialState
    gain_index=76;
  state SLOW
  state MGC
  state DECREASE_GAIN_AGC_Inner
    entry:
    gain_index = max(gain_index-AGC_G_dec_slow,0);
  state DoNothing
  state CHANGE_GAIN
    entry:
    gain_index = ManualGainIndex;
  state INCREASE_GAIN_Inner
    entry:
    gain_index = min(gain_index+AGC_G_inc_slow,76);
  state DECREASE_GAIN_AGC_Outer
    entry:
    gain_index = max(gain_index-AGC_G_dec_fast,0);
  state INCREASE_GAIN_Outer
    entry:
    gain_index = min(gain_index+AGC_G_inc_fast,76);
  state DECREASE_GAIN_ADC
    entry:
    gain_index = max(gain_index-ADC_G_dec_fast,0);
  state DECREASE_GAIN_LMT
    entry:
    gain_index = max(gain_index-LMT_G_dec_fast,0);
  (default) -> InitialState
  InitialState -> (junction 14) : after(T*1e-6,sec)
  (junction 14) -> MGC [order 2] : [mode==1]/{gain_index = ManualGainIndex;}
  (junction 14) -> SLOW [order 1] : [mode==0]
  MGC -> (junction 14) [order 2] : [mode==0]
  SLOW -> (junction 14) [order 1] : [mode==1]
  CHANGE_GAIN -> MGC : after(1e-7,sec)
  MGC -> CHANGE_GAIN [order 1] : [hasChanged(ManualGainIndex)]
  DECREASE_GAIN_LMT -> SLOW : after(C*1e-6,sec)
  SLOW -> DECREASE_GAIN_LMT [order 2] : at(N_LMT_H, LMT_H)
  DECREASE_GAIN_ADC -> SLOW : after(C*1e-6,sec)
  SLOW -> DECREASE_GAIN_ADC [order 3] : at(N_ADC_H, ADC_H)
  DECREASE_GAIN_AGC_Outer -> SLOW : after(C*1e-6,sec)
  SLOW -> DECREASE_GAIN_AGC_Outer [order 4] : at(1, POW_H_outer)
  DECREASE_GAIN_AGC_Inner -> SLOW : after(C*1e-6,sec)
  SLOW -> DECREASE_GAIN_AGC_Inner [order 5] : at(1, POW_H_inner)
  INCREASE_GAIN_Outer -> SLOW : after(C*1e-6,sec)
  SLOW -> INCREASE_GAIN_Outer [order 6] : at(1, POW_L_outer)
  INCREASE_GAIN_Inner -> SLOW : after(C*1e-6,sec)
  SLOW -> INCREASE_GAIN_Inner [order 7] : at(1, POW_L_inner)
  DoNothing -> SLOW
  SLOW -> DoNothing [order 8] : at(N_LMT_L, LMT_L)
  SLOW -> DoNothing [order 9] : at(N_ADC_L,ADC_L)
  data: mode input; N_LMT_H parameter double; N_LMT_L parameter double; N_ADC_H parameter double; N_ADC_L parameter double; gain_index output double; C parameter; ManualGainIndex input double; ADC_G_dec_fast parameter; AGC_G_inc_fast parameter; AGC_G_inc_slow parameter; LMT_G_dec_fast parameter; T parameter; AGC_G_dec_fast parameter; AGC_G_dec_slow parameter
  events: POW_L_outer input RISING_EDGE_EVENT; POW_L_inner input RISING_EDGE_EVENT; POW_H_inner input RISING_EDGE_EVENT; POW_H_outer input RISING_EDGE_EVENT; ADC_H input RISING_EDGE_EVENT; ADC_L input RISING_EDGE_EVENT; LMT_L input RISING_EDGE_EVENT; LMT_H input RISING_EDGE_EVENT; event input RISING_EDGE_EVENT

== matlab function QPSK_ad9361_radioIO_capture/QPSK Receiver1/Coarse Frequency Compensation/Find Frequency Offset/Find Frequency Offset ==
  data: N input; FreqOffset output; Tf input; FFTSig input; M parameter
function FreqOffset = findfreqoffset(N,Tf,FFTSig,M) %#codegen
%  Estimate frequency offset.
%  findfreqoffset(N,Tf,fvec,params) returns the estimated frequency offset
%  given time-domain frame length N, sample time vector Tf containing
%  [frameTime,offsetTime], complex FFT vector FFTsig, and modulation
%  order M.

% Find index of max magnitude, convert to offset symmetric about zero.
% Return a negative integer offset to be interpreted as a compensation.
[~,maxIdx] = max(FFTSig);
FFTSize = size(FFTSig,1);
if maxIdx > FFTSize/2
    OffsetIdx = FFTSize+1-maxIdx;
else
    OffsetIdx = 1-maxIdx;
end
% Map offset index to a frequency value.
% Compute offset using modulation alphabet size params.M.
Ts = Tf(1)/N; % Sample time
delta_f = 1/(Ts*FFTSize); % Frequency resolution of FFT
FreqOffset = OffsetIdx * delta_f / M;

== matlab function QPSK_ad9361_radioIO_capture/QPSK Receiver1/Data Decoding/Align Data ==
  data: Delay input; RxData input; Data output
function Data  = aligndata(Delay, RxData)
% Extract data from the buffered RxData, using the delay to find the frame 
% start
%
% Input:
% Delay - Index of frame start
% RxData - Buffered symbol-spaced data
% Output:
% Data - Data with the Barker code at frame start
%#codegen
Data = RxData(Delay+1:Delay+length(RxData)/2);

== matlab function QPSK_ad9361_radioIO_capture/QPSK Receiver1/Data Decoding/BitsToDecimal ==
  data: u input
function BitsToASCII(u)
% Convert bits to ASCII message.

coder.extrinsic('disp')

% Convert binary-valued column vector to 7-bit decimal values.
w = [64 32 16 8 4 2 1]; % binary digit weighting
Nbits = numel(u);
Ny = Nbits/7;
y = zeros(1,Ny);
for i = 0:Ny-1
    y(i+1) = w*u(7*i+(1:7));
end

% Display ASCII message to command window
disp(char(y));

== matlab function QPSK_ad9361_radioIO_capture/QPSK Receiver1/Data Decoding/Phase Offset Estimator/Phase Offset Detection ==
  data: In input; Out output
function Out = phasedecision(In)
% Map the estimated phase to one of -pi, -pi/2, 0, pi/2,  
%#codegen
% Out = round(In.*2./pi)./2.*pi;
% The above processing is equivalent to the following processing using
% if/else statements
%
% if In<pi/4 && In>-pi/4
%     Out = 0;
% elseif In>=pi/4 && In<pi*3/4
%     Out = pi/2;
% elseif In>=pi*3/4 || In<=-pi*3/4
%     Out = -pi;
% else
%     Out = -pi/2;
% end

if In<pi/4 && In>=-pi/4
    Out = 0;
elseif In>=pi/4 && In<pi*3/4
    Out = pi/2;
elseif In>=pi*3/4 || In<-pi*3/4
    Out = -pi;
else
    Out = -pi/2;
end

== matlab function QPSK_ad9361_radioIO_capture/QPSK Receiver1/Fine Frequency Compensation/PED ==
  data: In input; e output
function e = PED(In)
% Implementation of Maximum Likelihood Phase Error Detector listed in
% Chapter 7.2.2 of "Digital Communications - A Discrete-Time Approach" by
% Michael Rice. This employs a decision directed method.
% 
% Input: 
%   In - Input samples, oversampled by two
% Output:
%   e - Phase error, de
%#codegen

e = sign(real(In)).*imag(In) - sign(imag(In)).*real(In);

== matlab function QPSK_ad9361_radioIO_capture/QPSK Receiver1/Timing Recovery/Timing Recovery PLL/Interpolation Filter ==
  data: In input; Out output; mu input
function Out = interp_filter(In, mu)
% Prabolic piecewise polynomial interpolator, Farrow Interpolator with 
% alpha = 1/2, see Figure 8.4.16 of "Digital Communications - A 
% Discrete-Time Approach" by Michael Rice.
% Input:
%   In - Input samples, oversampled by two
%   mu - Difference between actual sampling instant and the optimal instant,
%        between zero and one
% Output:
%   Out - Interpolation output
%#codegen
persistent delay1 delay2 delay3; % Input delayed by 1, 2 and 3 samples
if isempty(delay1)
    [delay1, delay2, delay3] = deal(complex(0,0));
end

K = -0.5;

Out = delay2 + mu.*(K.*(In+delay2+delay3)+(1-K).*delay1)...
      + K.*(delay1+delay2-In-delay3).*mu.^2;
  
% Update delay buffers
delay3 = delay2;
delay2 = delay1;
delay1 = In;

== matlab function QPSK_ad9361_radioIO_capture/QPSK Receiver1/Timing Recovery/Timing Recovery PLL/NCO Control ==
  data: Delta input; Underflow output; mu output; sdrqpskrx parameter
function [Underflow, mu] = NCO_ctrl(Delta, sdrqpskrx)
% Implementation of modulo-1 counter for interpolation control listed in
% Figure 8.4.19 of "Digital Communications - A Discrete-Time Approach"
% by Michael Rice. See design details in Chapter 8.4.3 of the same book.
% 
% Input:
%   Delta - Loop filter output. If loop is in lock, delta would be small
%   qpsktxrx - Simulation parameter structure
% Output:
%   Underflow - Indicator of counter underflow. This is the strobe signal
%   for downstream processing
%   mu - Difference between actual sampling instant and the optimal instant,
%        between zero and one
%#codegen

% delay1 - Counter value delayed by 1 sample
% Regtemp - The estimated timing error normalized by half QPSK symbols
persistent delay1 Regtemp;  
if isempty(delay1)
    [delay1, Regtemp] = deal(0);
end
Upsampling = sdrqpskrx.Upsampling;
Downsampling = sdrqpskrx.Downsampling;
oversampling = Upsampling/Downsampling;

counter = mod(delay1,1)-Delta-1/oversampling; % decrementing counter
if counter < 0
    Underflow = 1;
    Regtemp = mod(delay1,1)/(Delta+1/oversampling);
else
    Underflow = 0;
end

mu = Regtemp;

% Update delay buffer
delay1 = mod(delay1,1)-Delta-1/oversampling;
